simulink model "MEEN_432_Proj1Part2"  (R2025a)
settings: Solver=ode45  StartTime=0.0  StopTime=25  FixedStep=1  RelTol=1e-3
values from neighbouring files (symbols this model uses):
  b1 = 1    [MEEN_432_Proj1Part2_Script.m]
  b2 = 1    [MEEN_432_Proj1Part2_Script.m]
  j1 = 100    [MEEN_432_Proj1Part2_Script.m]
  j2 = 1    [MEEN_432_Proj1Part2_Script.m]
  tau_applied = 10    [MEEN_432_Proj1Part2_Script.m]
  tau_load = 1    [MEEN_432_Proj1Part2_Script.m]
  w_0 = 0    [MEEN_432_Proj1Part2_Script.m]
settings Model: NumberOfSteps=100  Creator=caleb  LastModifiedBy=jr843

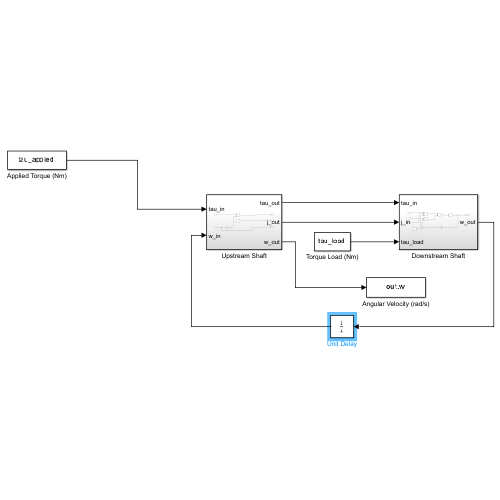
[thumbnail: Simulink's stored preview of the top-level diagram]
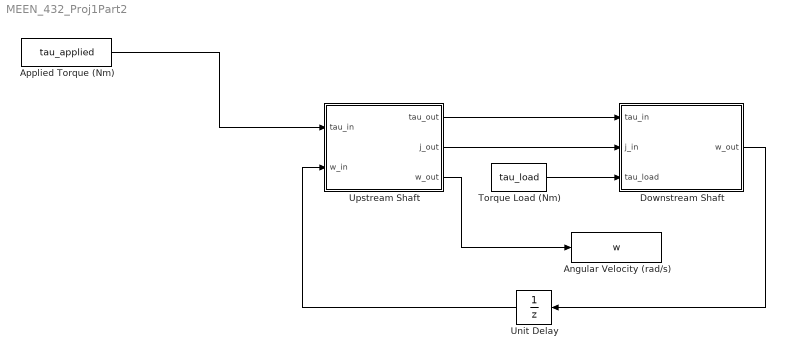
== system MEEN_432_Proj1Part2 ==
  Angular Velocity (rad/s) : ToWorkspace  VariableName=w  SaveFormat=Timeseries  SampleTime=-1
  Applied Torque (Nm) : Constant  Value=tau_applied
  Downstream Shaft : Subsystem
  Torque Load (Nm) : Constant  Value=tau_load
  Unit Delay : UnitDelay  InitialCondition=w_0  SampleTime=-1  HasFrameUpgradeWarning=on
  Upstream Shaft : Subsystem
  wires:
  Applied Torque (Nm)/1 -> Upstream Shaft/1(tau_in)
  Upstream Shaft/1(tau_out) -> Downstream Shaft/1(tau_in)
  Upstream Shaft/2(j_out) -> Downstream Shaft/2(j_in)
  Downstream Shaft/1(w_out) -> Unit Delay/1
  Unit Delay/1 -> Upstream Shaft/2(w_in)
  Torque Load (Nm)/1 -> Downstream Shaft/3(tau_load)
  Upstream Shaft/3(w_out) -> Angular Velocity (rad/s)/1

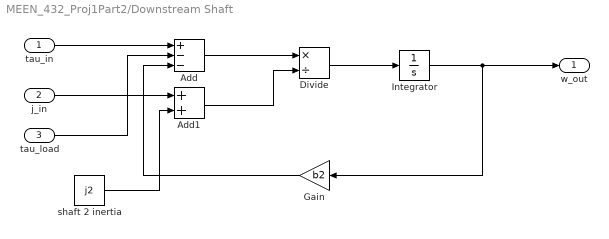
== system MEEN_432_Proj1Part2/Downstream Shaft ==
  tau_in : Inport
  j_in : Inport  Port=2
  tau_load : Inport  Port=3
  Add : Sum  Inputs=+--
  Add1 : Sum
  Divide : Product  Inputs=*/
  Gain : Gain  Gain=b2
  Integrator : Integrator
  shaft 2 inertia : Constant  Value=j2
  w_out : Outport
  wires:
  tau_in/1 -> Add/1
  tau_load/1 -> Add/2
  shaft 2 inertia/1 -> Add1/2
  j_in/1 -> Add1/1
  Add/1 -> Divide/1
  Add1/1 -> Divide/2
  Divide/1 -> Integrator/1
  Integrator/1 -> w_out/1, Gain/1
  Gain/1 -> Add/3

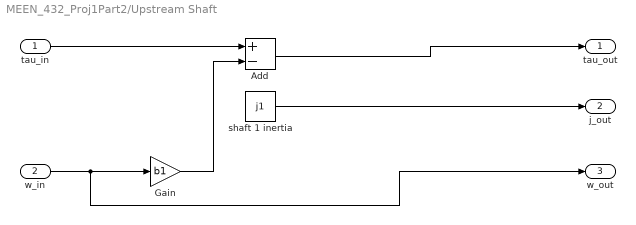
== system MEEN_432_Proj1Part2/Upstream Shaft ==
  tau_in : Inport
  w_in : Inport  Port=2
  Add : Sum  Inputs=+-
  Gain : Gain  Gain=b1
  shaft 1 inertia : Constant  Value=j1
  tau_out : Outport
  j_out : Outport  Port=2
  w_out : Outport  Port=3
  wires:
  tau_in/1 -> Add/1
  w_in/1 -> w_out/1, Gain/1
  Gain/1 -> Add/2
  Add/1 -> tau_out/1
  shaft 1 inertia/1 -> j_out/1
